simulink model "sim_SMC_algorithm"  (R2024b)
settings: Solver=FixedStepAuto  StartTime=0.0  StopTime=10.0  FixedStep=Tsim  RelTol=1e-3
InitFcn:
  | Tsim = 1e-4;
settings Model: Creator=Thu  LastModifiedBy=Lenovo
settings RTWCC: GPUComputeCapability=3.5

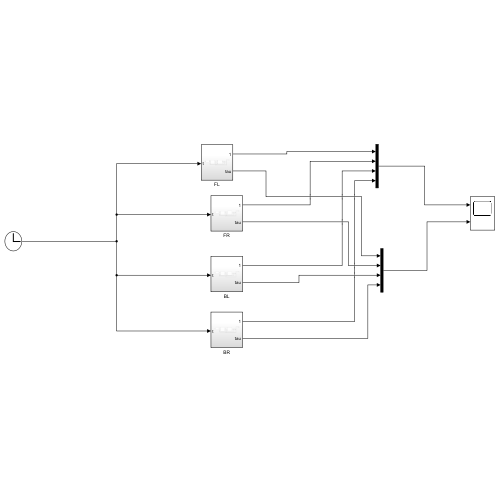
[thumbnail: Simulink's stored preview of the top-level diagram]
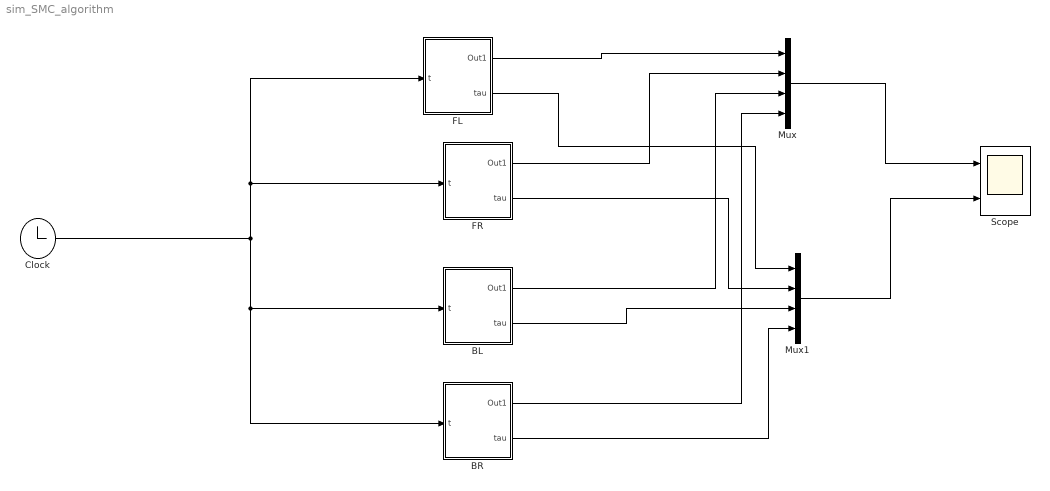
== system sim_SMC_algorithm ==
  BL : Subsystem
  BR : Subsystem
  Clock : Clock
  FL : Subsystem
  FR : Subsystem
  Mux : Mux
  Mux1 : Mux
  Scope : Scope  NumInputPorts=2
  wires:
  Clock/1 -> BR/1(t), BL/1(t), FR/1(t), FL/1(t)
  BR/1(Out1) -> Mux/4
  BR/2(tau) -> Mux1/4
  FL/1(Out1) -> Mux/1
  FR/1(Out1) -> Mux/2
  BL/1(Out1) -> Mux/3
  Mux/1 -> Scope/1
  FL/2(tau) -> Mux1/1
  FR/2(tau) -> Mux1/2
  BL/2(tau) -> Mux1/3
  Mux1/1 -> Scope/2

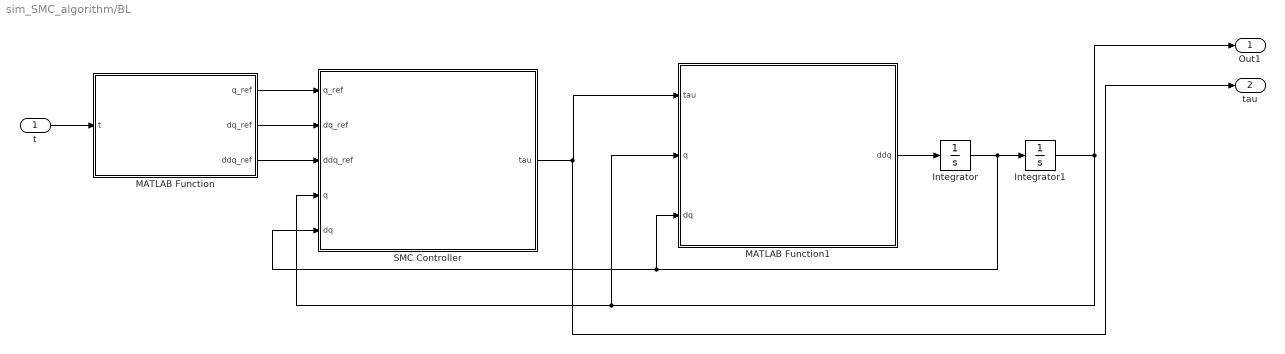
== system sim_SMC_algorithm/BL ==
  t : Inport
  Integrator : Integrator  InitialCondition=[0; 0]
  Integrator1 : Integrator  InitialCondition=[0.727; -1.78]
  MATLAB Function : MATLAB Function  TreatAsAtomicUnit=on
  MATLAB Function1 : MATLAB Function  TreatAsAtomicUnit=on
  SMC Controller : MATLAB Function  TreatAsAtomicUnit=on
  Out1 : Outport
  tau : Outport  Port=2
  wires:
  MATLAB Function/1(q_ref) -> SMC Controller/1(q_ref)
  MATLAB Function/3(ddq_ref) -> SMC Controller/3(ddq_ref)
  Integrator/1 -> Integrator1/1, SMC Controller/5(dq), MATLAB Function1/3(dq)
  MATLAB Function1/1(ddq) -> Integrator/1
  SMC Controller/1(tau) -> tau/1, MATLAB Function1/1(tau)
  MATLAB Function/2(dq_ref) -> SMC Controller/2(dq_ref)
  t/1 -> MATLAB Function/1(t)
  Integrator1/1 -> Out1/1, MATLAB Function1/2(q), SMC Controller/4(q)

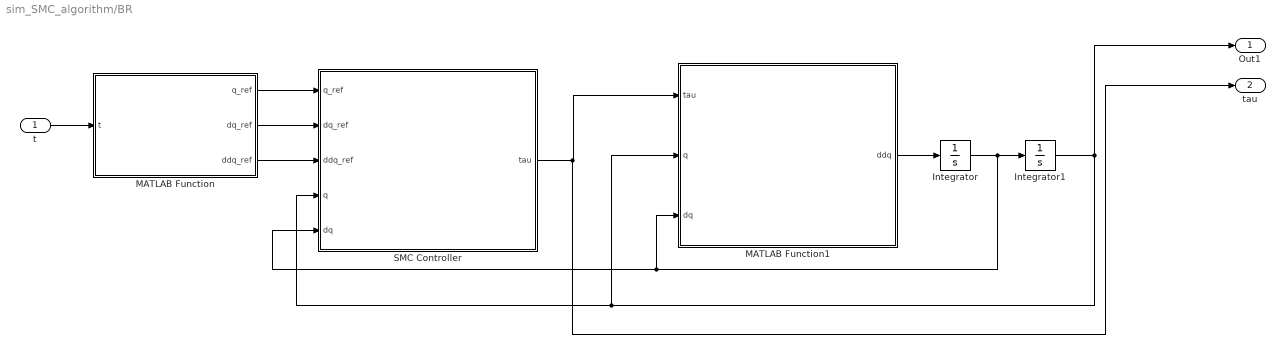
== system sim_SMC_algorithm/BR ==
  t : Inport
  Integrator : Integrator  InitialCondition=[0; 0]
  Integrator1 : Integrator  InitialCondition=[1.02; -1.78]
  MATLAB Function : MATLAB Function  TreatAsAtomicUnit=on
  MATLAB Function1 : MATLAB Function  TreatAsAtomicUnit=on
  SMC Controller : MATLAB Function  TreatAsAtomicUnit=on
  Out1 : Outport
  tau : Outport  Port=2
  wires:
  Integrator1/1 -> Out1/1, SMC Controller/4(q), MATLAB Function1/2(q)
  t/1 -> MATLAB Function/1(t)
  MATLAB Function/2(dq_ref) -> SMC Controller/2(dq_ref)
  SMC Controller/1(tau) -> MATLAB Function1/1(tau), tau/1
  MATLAB Function1/1(ddq) -> Integrator/1
  Integrator/1 -> MATLAB Function1/3(dq), SMC Controller/5(dq), Integrator1/1
  MATLAB Function/3(ddq_ref) -> SMC Controller/3(ddq_ref)
  MATLAB Function/1(q_ref) -> SMC Controller/1(q_ref)

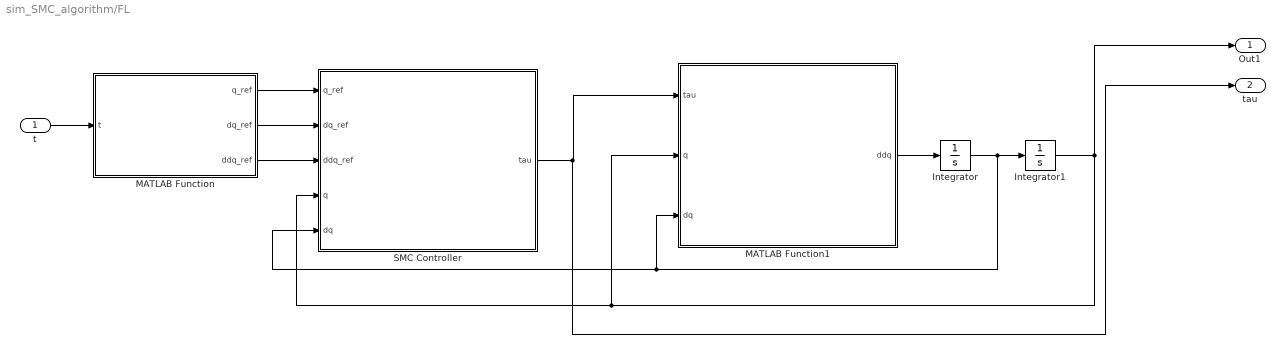
== system sim_SMC_algorithm/FL ==
  t : Inport
  Integrator : Integrator  InitialCondition=[0; 0]
  Integrator1 : Integrator  InitialCondition=[1.02; -1.78]
  MATLAB Function : MATLAB Function  TreatAsAtomicUnit=on
  MATLAB Function1 : MATLAB Function  TreatAsAtomicUnit=on
  SMC Controller : MATLAB Function  TreatAsAtomicUnit=on
  Out1 : Outport
  tau : Outport  Port=2
  wires:
  Integrator1/1 -> Out1/1, MATLAB Function1/2(q), SMC Controller/4(q)
  MATLAB Function/1(q_ref) -> SMC Controller/1(q_ref)
  MATLAB Function/3(ddq_ref) -> SMC Controller/3(ddq_ref)
  Integrator/1 -> Integrator1/1, SMC Controller/5(dq), MATLAB Function1/3(dq)
  MATLAB Function1/1(ddq) -> Integrator/1
  SMC Controller/1(tau) -> tau/1, MATLAB Function1/1(tau)
  MATLAB Function/2(dq_ref) -> SMC Controller/2(dq_ref)
  t/1 -> MATLAB Function/1(t)

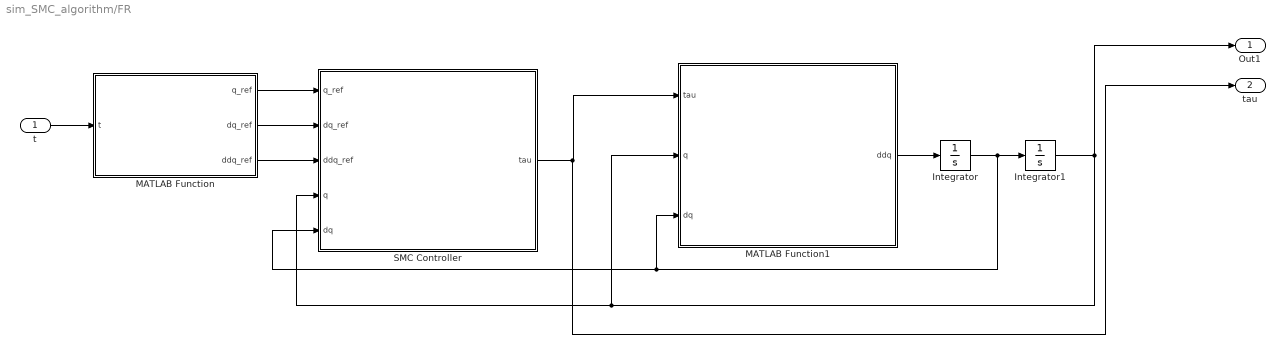
== system sim_SMC_algorithm/FR ==
  t : Inport
  Integrator : Integrator  InitialCondition=[0; 0]
  Integrator1 : Integrator  InitialCondition=[0.727; -1.78]
  MATLAB Function : MATLAB Function  TreatAsAtomicUnit=on
  MATLAB Function1 : MATLAB Function  TreatAsAtomicUnit=on
  SMC Controller : MATLAB Function  TreatAsAtomicUnit=on
  Out1 : Outport
  tau : Outport  Port=2
  wires:
  t/1 -> MATLAB Function/1(t)
  MATLAB Function/2(dq_ref) -> SMC Controller/2(dq_ref)
  SMC Controller/1(tau) -> MATLAB Function1/1(tau), tau/1
  MATLAB Function1/1(ddq) -> Integrator/1
  Integrator/1 -> MATLAB Function1/3(dq), SMC Controller/5(dq), Integrator1/1
  MATLAB Function/3(ddq_ref) -> SMC Controller/3(ddq_ref)
  MATLAB Function/1(q_ref) -> SMC Controller/1(q_ref)
  Integrator1/1 -> Out1/1, SMC Controller/4(q), MATLAB Function1/2(q)

== matlab function sim_SMC_algorithm/BR/MATLAB Function ==
  data: t input; q_ref output; dq_ref output; ddq_ref output
function [q_ref, dq_ref, ddq_ref] = gait_planner_Trot(t)
    % ÉP KIỂU ĐẦU RA [2x1]
    q_ref = zeros(2,1); dq_ref = zeros(2,1); ddq_ref = zeros(2,1);

    % =======================================================
    % KHAI BÁO ĐỘ LỆCH PHA (OFFSET)
    % - Chân FL và BR: offset = 0.0
    % - Chân FR và BL: offset = 0.5 (Lệch nửa chu kỳ)
    % =======================================================
    offset = 0.0; 
    
    % 1. Tính vị trí hiện tại
    q_ref = calc_IK(t, offset);
    
    % 2. Tự động tính Đạo hàm (Vận tốc, Gia tốc) bên trong hàm
    % Dùng khoảng thời gian cực nhỏ dt để nội suy đạo hàm
    dt = 1e-3; 
    q_prev = calc_IK(t - dt, offset);
    q_prev2 = calc_IK(t - 2*dt, offset);
    
    dq_ref = (q_ref - q_prev) / dt;
    ddq_ref = (q_ref - 2*q_prev + q_prev2) / (dt^2);
    
    % Giới hạn gia tốc để tránh giật vọt (Spike) lúc chạm đất
    ddq_ref = max(min(ddq_ref, 50), -50); 
end

% HÀM CON: GIẢI ĐỘNG HỌC NGHỊCH (Bê nguyên từ GaitPlanner.hpp)
function q = calc_IK(t, offset)
    T_cycle = 1.0; S = 0.08; H = 0.01; y0 = -0.25;
    L1 = 0.2; L2 = 0.2;
    
    theta = (t / T_cycle + offset) * 2 * pi;
    theta_mod = mod(theta, 2 * pi);
    
    % Tạo hình bán elip
    if theta_mod < pi
        x = (S / 2.0) * cos(theta_mod);
        y = y0 + H * sin(theta_mod);
    else
        x = -(S / 2.0) * cos(theta_mod - pi);
        y = y0;
    end
    
    % Giới hạn vùng không gian làm việc (Workspace)
    L_sq = x^2 + y^2;
    max_reach = L1 + L2 - 0.001;
    if L_sq > max_reach^2
        scale = max_reach / sqrt(L_sq);
        x = x * scale; y = y * scale;
        L_sq = x^2 + y^2;
    end
    
    % Giải Inverse Kinematics
    cos_q2 = (L_sq - L1^2 - L2^2) / (2 * L1 * L2);
    cos_q2 = max(min(cos_q2, 1.0), -1.0);
    q2 = -acos(cos_q2);
    
    alpha = atan2(y, x);
    beta = atan2(L2 * sin(q2), L1 + L2 * cos(q2));
    q1 = (alpha - beta) + pi / 2.0;
    
    q = [q1; q2];
end

== matlab function sim_SMC_algorithm/BR/MATLAB Function1 ==
  data: tau input; ddq output; q input; dq input
function ddq = dynamics_plant(tau, q, dq)
% 1. KHỞI TẠO KÍCH THƯỚC ĐẦU RA 
    ddq = zeros(2,1);

% ÉP KIỂU VECTOR CỘT
    tau = tau(:); q = q(:); dq = dq(:);
    
    q1 = q(1); q2 = q(2);
    dq1 = dq(1); dq2 = dq(2);

    % Ma trận Động lực học (Giữ nguyên như bên SMC)
    M = [cos(q2)/50 + 0.040128, cos(q2)/100 + 0.0066948;
         cos(q2)/100 + 0.0066948, 0.0066948];
         
    C = [dq2*sin(q2)*(-0.01),     sin(q2)*(dq1 + dq2)*(-0.01);
         (dq1*sin(q2))/100,       0];
         
    G = [cos(q1+q2)*0.4905 + cos(q1)*1.962;
         cos(q1+q2)*0.4905];

    % Giải phương trình động lực học tìm gia tốc thực tế
    % Dùng toán tử "\" (mldivide) của MATLAB thay cho inv(M) để hệ thống tính toán ổn định và nhanh hơn
    ddq = M \ (tau - C*dq - G); 
end

== matlab function sim_SMC_algorithm/BR/SMC Controller ==
  data: q_ref input; tau output; dq_ref input; ddq_ref input; q input; dq input
function tau = SMC_controller(q_ref, dq_ref, ddq_ref, q, dq)
% 1. KHỞI TẠO KÍCH THƯỚC ĐẦU RA
    tau = zeros(2,1);    
    
% ÉP KIỂU VECTOR CỘT [2x1] (Cực kỳ quan trọng trong Simulink)
    q_ref = q_ref(:); dq_ref = dq_ref(:); ddq_ref = ddq_ref(:);
    q = q(:); dq = dq(:);

    %% 1. Các thông số bộ điều khiển 
    lambda = [100 0; 0 100]; % Ma trận hệ số mặt trượt
    K = [15 0; 0 8];        % Độ lợi điều khiển 
    Phi = [3.0 0; 0 3.0];  % Bề dày lớp biên để chống rung 

    q1 = q(1); q2 = q(2);
    dq1 = dq(1); dq2 = dq(2);

    %% 2. Tính toán Ma trận Động lực học 
    M = [cos(q2)/50 + 0.040128, cos(q2)/100 + 0.0066948;
         cos(q2)/100 + 0.0066948, 0.0066948];

    C = [dq2*sin(q2)*(-0.01),     sin(q2)*(dq1 + dq2)*(-0.01);
         (dq1*sin(q2))/100,       0];

    G = [cos(q1+q2)*0.4905 + cos(q1)*1.962;
         cos(q1+q2)*0.4905];

    %% 3. Thuật toán SMC
    e = q - q_ref;      % Sai số vị trí
    de = dq - dq_ref;   % Sai số vận tốc
    s = de + lambda * e;

    % Điều khiển tương đương 
    tau_eq = M * (ddq_ref - lambda * de) + C * dq + G;

    % Điều khiển chuyển mạch (Dùng hàm Saturation vector hóa)
    phi_diag = diag(Phi); % Trích xuất phần tử đường chéo [0.1; 0.1]
    sat_s = max(min(s ./ phi_diag, 1), -1); % Ràng buộc giá trị trong khoảng [-1, 1]

    tau_reach = -M * K * sat_s;

    %% 4. Đầu ra mô-men xoắn
    tau = tau_eq + tau_reach;
end

== matlab function sim_SMC_algorithm/FL/MATLAB Function1 ==
  data: tau input; ddq output; q input; dq input
function ddq = dynamics_plant(tau, q, dq)
% 1. KHỞI TẠO KÍCH THƯỚC ĐẦU RA 
    ddq = zeros(2,1);

% ÉP KIỂU VECTOR CỘT
    tau = tau(:); q = q(:); dq = dq(:);
    
    q1 = q(1); q2 = q(2);
    dq1 = dq(1); dq2 = dq(2);

    % Ma trận Động lực học (Giữ nguyên như bên SMC)
    M = [cos(q2)/50 + 0.040128, cos(q2)/100 + 0.0066948;
         cos(q2)/100 + 0.0066948, 0.0066948];
         
    C = [dq2*sin(q2)*(-0.01),     sin(q2)*(dq1 + dq2)*(-0.01);
         (dq1*sin(q2))/100,       0];
         
    G = [cos(q1+q2)*0.4905 + cos(q1)*1.962;
         cos(q1+q2)*0.4905];

    % Giải phương trình động lực học tìm gia tốc thực tế
    % Dùng toán tử "\" (mldivide) của MATLAB thay cho inv(M) để hệ thống tính toán ổn định và nhanh hơn
    ddq = M \ (tau - C*dq - G); 
end

== matlab function sim_SMC_algorithm/FL/SMC Controller ==
  data: q_ref input; tau output; dq_ref input; ddq_ref input; q input; dq input
function tau = SMC_controller(q_ref, dq_ref, ddq_ref, q, dq)
% 1. KHỞI TẠO KÍCH THƯỚC ĐẦU RA
    tau = zeros(2,1);    
    
% ÉP KIỂU VECTOR CỘT [2x1] (Cực kỳ quan trọng trong Simulink)
    q_ref = q_ref(:); dq_ref = dq_ref(:); ddq_ref = ddq_ref(:);
    q = q(:); dq = dq(:);

    %% 1. Các thông số bộ điều khiển 
    lambda = [100 0; 0 100]; % Ma trận hệ số mặt trượt
    K = [15 0; 0 8];        % Độ lợi điều khiển 
    Phi = [3.0 0; 0 3.0];  % Bề dày lớp biên để chống rung 

    q1 = q(1); q2 = q(2);
    dq1 = dq(1); dq2 = dq(2);

    %% 2. Tính toán Ma trận Động lực học 
    M = [cos(q2)/50 + 0.040128, cos(q2)/100 + 0.0066948;
         cos(q2)/100 + 0.0066948, 0.0066948];

    C = [dq2*sin(q2)*(-0.01),     sin(q2)*(dq1 + dq2)*(-0.01);
         (dq1*sin(q2))/100,       0];

    G = [cos(q1+q2)*0.4905 + cos(q1)*1.962;
         cos(q1+q2)*0.4905];

    %% 3. Thuật toán SMC
    e = q - q_ref;      % Sai số vị trí
    de = dq - dq_ref;   % Sai số vận tốc
    s = de + lambda * e;

    % Điều khiển tương đương 
    tau_eq = M * (ddq_ref - lambda * de) + C * dq + G;

    % Điều khiển chuyển mạch (Dùng hàm Saturation vector hóa)
    phi_diag = diag(Phi); % Trích xuất phần tử đường chéo [0.1; 0.1]
    sat_s = max(min(s ./ phi_diag, 1), -1); % Ràng buộc giá trị trong khoảng [-1, 1]

    tau_reach = -M * K * sat_s;

    %% 4. Đầu ra mô-men xoắn
    tau = tau_eq + tau_reach;
end

== matlab function sim_SMC_algorithm/FL/MATLAB Function ==
  data: t input; q_ref output; dq_ref output; ddq_ref output
function [q_ref, dq_ref, ddq_ref] = gait_planner_Trot(t)
    % ÉP KIỂU ĐẦU RA [2x1]
    q_ref = zeros(2,1); dq_ref = zeros(2,1); ddq_ref = zeros(2,1);

    % =======================================================
    % KHAI BÁO ĐỘ LỆCH PHA (OFFSET)
    % - Chân FL và BR: offset = 0.0
    % - Chân FR và BL: offset = 0.5 (Lệch nửa chu kỳ)
    % =======================================================
    offset = 0.0; 
    
    % 1. Tính vị trí hiện tại
    q_ref = calc_IK(t, offset);
    
    % 2. Tự động tính Đạo hàm (Vận tốc, Gia tốc) bên trong hàm
    % Dùng khoảng thời gian cực nhỏ dt để nội suy đạo hàm
    dt = 1e-3; 
    q_prev = calc_IK(t - dt, offset);
    q_prev2 = calc_IK(t - 2*dt, offset);
    
    dq_ref = (q_ref - q_prev) / dt;
    ddq_ref = (q_ref - 2*q_prev + q_prev2) / (dt^2);
    
    % Giới hạn gia tốc để tránh giật vọt (Spike) lúc chạm đất
    ddq_ref = max(min(ddq_ref, 50), -50); 
end

% HÀM CON: GIẢI ĐỘNG HỌC NGHỊCH (Bê nguyên từ GaitPlanner.hpp)
function q = calc_IK(t, offset)
    T_cycle = 1.0; S = 0.08; H = 0.01; y0 = -0.25;
    L1 = 0.2; L2 = 0.2;
    
    theta = (t / T_cycle + offset) * 2 * pi;
    theta_mod = mod(theta, 2 * pi);
    
    % Tạo hình bán elip
    if theta_mod < pi
        x = (S / 2.0) * cos(theta_mod);
        y = y0 + H * sin(theta_mod);
    else
        x = -(S / 2.0) * cos(theta_mod - pi);
        y = y0;
    end
    
    % Giới hạn vùng không gian làm việc (Workspace)
    L_sq = x^2 + y^2;
    max_reach = L1 + L2 - 0.001;
    if L_sq > max_reach^2
        scale = max_reach / sqrt(L_sq);
        x = x * scale; y = y * scale;
        L_sq = x^2 + y^2;
    end
    
    % Giải Inverse Kinematics
    cos_q2 = (L_sq - L1^2 - L2^2) / (2 * L1 * L2);
    cos_q2 = max(min(cos_q2, 1.0), -1.0);
    q2 = -acos(cos_q2);
    
    alpha = atan2(y, x);
    beta = atan2(L2 * sin(q2), L1 + L2 * cos(q2));
    q1 = (alpha - beta) + pi / 2.0;
    
    q = [q1; q2];
end

== matlab function sim_SMC_algorithm/FR/MATLAB Function ==
  data: t input; q_ref output; dq_ref output; ddq_ref output
function [q_ref, dq_ref, ddq_ref] = gait_planner_Trot(t)
    % ÉP KIỂU ĐẦU RA [2x1]
    q_ref = zeros(2,1); dq_ref = zeros(2,1); ddq_ref = zeros(2,1);

    % =======================================================
    % KHAI BÁO ĐỘ LỆCH PHA (OFFSET)
    % - Chân FL và BR: offset = 0.0
    % - Chân FR và BL: offset = 0.5 (Lệch nửa chu kỳ)
    % =======================================================
    offset = 0.5; 
    
    % 1. Tính vị trí hiện tại
    q_ref = calc_IK(t, offset);
    
    % 2. Tự động tính Đạo hàm (Vận tốc, Gia tốc) bên trong hàm
    % Dùng khoảng thời gian cực nhỏ dt để nội suy đạo hàm
    dt = 1e-3; 
    q_prev = calc_IK(t - dt, offset);
    q_prev2 = calc_IK(t - 2*dt, offset);
    
    dq_ref = (q_ref - q_prev) / dt;
    ddq_ref = (q_ref - 2*q_prev + q_prev2) / (dt^2);
    
    % Giới hạn gia tốc để tránh giật vọt (Spike) lúc chạm đất
    ddq_ref = max(min(ddq_ref, 50), -50); 
end

% HÀM CON: GIẢI ĐỘNG HỌC NGHỊCH (Bê nguyên từ GaitPlanner.hpp)
function q = calc_IK(t, offset)
    T_cycle = 1.0; S = 0.08; H = 0.01; y0 = -0.25;
    L1 = 0.2; L2 = 0.2;
    
    theta = (t / T_cycle + offset) * 2 * pi;
    theta_mod = mod(theta, 2 * pi);
    
    % Tạo hình bán elip
    if theta_mod < pi
        x = (S / 2.0) * cos(theta_mod);
        y = y0 + H * sin(theta_mod);
    else
        x = -(S / 2.0) * cos(theta_mod - pi);
        y = y0;
    end
    
    % Giới hạn vùng không gian làm việc (Workspace)
    L_sq = x^2 + y^2;
    max_reach = L1 + L2 - 0.001;
    if L_sq > max_reach^2
        scale = max_reach / sqrt(L_sq);
        x = x * scale; y = y * scale;
        L_sq = x^2 + y^2;
    end
    
    % Giải Inverse Kinematics
    cos_q2 = (L_sq - L1^2 - L2^2) / (2 * L1 * L2);
    cos_q2 = max(min(cos_q2, 1.0), -1.0);
    q2 = -acos(cos_q2);
    
    alpha = atan2(y, x);
    beta = atan2(L2 * sin(q2), L1 + L2 * cos(q2));
    q1 = (alpha - beta) + pi / 2.0;
    
    q = [q1; q2];
end

== matlab function sim_SMC_algorithm/FR/MATLAB Function1 ==
  data: tau input; ddq output; q input; dq input
function ddq = dynamics_plant(tau, q, dq)
% 1. KHỞI TẠO KÍCH THƯỚC ĐẦU RA 
    ddq = zeros(2,1);

% ÉP KIỂU VECTOR CỘT
    tau = tau(:); q = q(:); dq = dq(:);
    
    q1 = q(1); q2 = q(2);
    dq1 = dq(1); dq2 = dq(2);

    % Ma trận Động lực học (Giữ nguyên như bên SMC)
    M = [cos(q2)/50 + 0.040128, cos(q2)/100 + 0.0066948;
         cos(q2)/100 + 0.0066948, 0.0066948];
         
    C = [dq2*sin(q2)*(-0.01),     sin(q2)*(dq1 + dq2)*(-0.01);
         (dq1*sin(q2))/100,       0];
         
    G = [cos(q1+q2)*0.4905 + cos(q1)*1.962;
         cos(q1+q2)*0.4905];

    % Giải phương trình động lực học tìm gia tốc thực tế
    % Dùng toán tử "\" (mldivide) của MATLAB thay cho inv(M) để hệ thống tính toán ổn định và nhanh hơn
    ddq = M \ (tau - C*dq - G); 
end

== matlab function sim_SMC_algorithm/FR/SMC Controller ==
  data: q_ref input; tau output; dq_ref input; ddq_ref input; q input; dq input
function tau = SMC_controller(q_ref, dq_ref, ddq_ref, q, dq)
% 1. KHỞI TẠO KÍCH THƯỚC ĐẦU RA
    tau = zeros(2,1);    
    
% ÉP KIỂU VECTOR CỘT [2x1] (Cực kỳ quan trọng trong Simulink)
    q_ref = q_ref(:); dq_ref = dq_ref(:); ddq_ref = ddq_ref(:);
    q = q(:); dq = dq(:);

    %% 1. Các thông số bộ điều khiển 
    lambda = [100 0; 0 100]; % Ma trận hệ số mặt trượt
    K = [15 0; 0 8];        % Độ lợi điều khiển 
    Phi = [3.0 0; 0 3.0];  % Bề dày lớp biên để chống rung 

    q1 = q(1); q2 = q(2);
    dq1 = dq(1); dq2 = dq(2);

    %% 2. Tính toán Ma trận Động lực học 
    M = [cos(q2)/50 + 0.040128, cos(q2)/100 + 0.0066948;
         cos(q2)/100 + 0.0066948, 0.0066948];

    C = [dq2*sin(q2)*(-0.01),     sin(q2)*(dq1 + dq2)*(-0.01);
         (dq1*sin(q2))/100,       0];

    G = [cos(q1+q2)*0.4905 + cos(q1)*1.962;
         cos(q1+q2)*0.4905];

    %% 3. Thuật toán SMC
    e = q - q_ref;      % Sai số vị trí
    de = dq - dq_ref;   % Sai số vận tốc
    s = de + lambda * e;

    % Điều khiển tương đương 
    tau_eq = M * (ddq_ref - lambda * de) + C * dq + G;

    % Điều khiển chuyển mạch (Dùng hàm Saturation vector hóa)
    phi_diag = diag(Phi); % Trích xuất phần tử đường chéo [0.1; 0.1]
    sat_s = max(min(s ./ phi_diag, 1), -1); % Ràng buộc giá trị trong khoảng [-1, 1]

    tau_reach = -M * K * sat_s;

    %% 4. Đầu ra mô-men xoắn
    tau = tau_eq + tau_reach;
end

== matlab function sim_SMC_algorithm/BL/MATLAB Function ==
  data: t input; q_ref output; dq_ref output; ddq_ref output
function [q_ref, dq_ref, ddq_ref] = gait_planner_Trot(t)
    % ÉP KIỂU ĐẦU RA [2x1]
    q_ref = zeros(2,1); dq_ref = zeros(2,1); ddq_ref = zeros(2,1);

    % =======================================================
    % KHAI BÁO ĐỘ LỆCH PHA (OFFSET)
    % - Chân FL và BR: offset = 0.0
    % - Chân FR và BL: offset = 0.5 (Lệch nửa chu kỳ)
    % =======================================================
    offset = 0.5; 
    
    % 1. Tính vị trí hiện tại
    q_ref = calc_IK(t, offset);
    
    % 2. Tự động tính Đạo hàm (Vận tốc, Gia tốc) bên trong hàm
    % Dùng khoảng thời gian cực nhỏ dt để nội suy đạo hàm
    dt = 1e-3; 
    q_prev = calc_IK(t - dt, offset);
    q_prev2 = calc_IK(t - 2*dt, offset);
    
    dq_ref = (q_ref - q_prev) / dt;
    ddq_ref = (q_ref - 2*q_prev + q_prev2) / (dt^2);
    
    % Giới hạn gia tốc để tránh giật vọt (Spike) lúc chạm đất
    ddq_ref = max(min(ddq_ref, 50), -50); 
end

% HÀM CON: GIẢI ĐỘNG HỌC NGHỊCH (Bê nguyên từ GaitPlanner.hpp)
function q = calc_IK(t, offset)
    T_cycle = 1.0; S = 0.08; H = 0.01; y0 = -0.25;
    L1 = 0.2; L2 = 0.2;
    
    theta = (t / T_cycle + offset) * 2 * pi;
    theta_mod = mod(theta, 2 * pi);
    
    % Tạo hình bán elip
    if theta_mod < pi
        x = (S / 2.0) * cos(theta_mod);
        y = y0 + H * sin(theta_mod);
    else
        x = -(S / 2.0) * cos(theta_mod - pi);
        y = y0;
    end
    
    % Giới hạn vùng không gian làm việc (Workspace)
    L_sq = x^2 + y^2;
    max_reach = L1 + L2 - 0.001;
    if L_sq > max_reach^2
        scale = max_reach / sqrt(L_sq);
        x = x * scale; y = y * scale;
        L_sq = x^2 + y^2;
    end
    
    % Giải Inverse Kinematics
    cos_q2 = (L_sq - L1^2 - L2^2) / (2 * L1 * L2);
    cos_q2 = max(min(cos_q2, 1.0), -1.0);
    q2 = -acos(cos_q2);
    
    alpha = atan2(y, x);
    beta = atan2(L2 * sin(q2), L1 + L2 * cos(q2));
    q1 = (alpha - beta) + pi / 2.0;
    
    q = [q1; q2];
end

== matlab function sim_SMC_algorithm/BL/MATLAB Function1 ==
  data: tau input; ddq output; q input; dq input
function ddq = dynamics_plant(tau, q, dq)
% 1. KHỞI TẠO KÍCH THƯỚC ĐẦU RA 
    ddq = zeros(2,1);

% ÉP KIỂU VECTOR CỘT
    tau = tau(:); q = q(:); dq = dq(:);
    
    q1 = q(1); q2 = q(2);
    dq1 = dq(1); dq2 = dq(2);

    % Ma trận Động lực học (Giữ nguyên như bên SMC)
    M = [cos(q2)/50 + 0.040128, cos(q2)/100 + 0.0066948;
         cos(q2)/100 + 0.0066948, 0.0066948];
         
    C = [dq2*sin(q2)*(-0.01),     sin(q2)*(dq1 + dq2)*(-0.01);
         (dq1*sin(q2))/100,       0];
         
    G = [cos(q1+q2)*0.4905 + cos(q1)*1.962;
         cos(q1+q2)*0.4905];

    % Giải phương trình động lực học tìm gia tốc thực tế
    % Dùng toán tử "\" (mldivide) của MATLAB thay cho inv(M) để hệ thống tính toán ổn định và nhanh hơn
    ddq = M \ (tau - C*dq - G); 
end

== matlab function sim_SMC_algorithm/BL/SMC Controller ==
  data: q_ref input; tau output; dq_ref input; ddq_ref input; q input; dq input
function tau = SMC_controller(q_ref, dq_ref, ddq_ref, q, dq)
% 1. KHỞI TẠO KÍCH THƯỚC ĐẦU RA
    tau = zeros(2,1);    
    
% ÉP KIỂU VECTOR CỘT [2x1] (Cực kỳ quan trọng trong Simulink)
    q_ref = q_ref(:); dq_ref = dq_ref(:); ddq_ref = ddq_ref(:);
    q = q(:); dq = dq(:);

    %% 1. Các thông số bộ điều khiển 
    lambda = [100 0; 0 100]; % Ma trận hệ số mặt trượt
    K = [15 0; 0 8];        % Độ lợi điều khiển 
    Phi = [3.0 0; 0 3.0];  % Bề dày lớp biên để chống rung 

    q1 = q(1); q2 = q(2);
    dq1 = dq(1); dq2 = dq(2);

    %% 2. Tính toán Ma trận Động lực học 
    M = [cos(q2)/50 + 0.040128, cos(q2)/100 + 0.0066948;
         cos(q2)/100 + 0.0066948, 0.0066948];

    C = [dq2*sin(q2)*(-0.01),     sin(q2)*(dq1 + dq2)*(-0.01);
         (dq1*sin(q2))/100,       0];

    G = [cos(q1+q2)*0.4905 + cos(q1)*1.962;
         cos(q1+q2)*0.4905];

    %% 3. Thuật toán SMC
    e = q - q_ref;      % Sai số vị trí
    de = dq - dq_ref;   % Sai số vận tốc
    s = de + lambda * e;

    % Điều khiển tương đương 
    tau_eq = M * (ddq_ref - lambda * de) + C * dq + G;

    % Điều khiển chuyển mạch (Dùng hàm Saturation vector hóa)
    phi_diag = diag(Phi); % Trích xuất phần tử đường chéo [0.1; 0.1]
    sat_s = max(min(s ./ phi_diag, 1), -1); % Ràng buộc giá trị trong khoảng [-1, 1]

    tau_reach = -M * K * sat_s;

    %% 4. Đầu ra mô-men xoắn
    tau = tau_eq + tau_reach;
end
